simulink subsystem "accelerometer"  (R2023b)
settings: Solver=VariableStepAuto  StartTime=0.0  StopTime=10.0  RelTol=1e-3
undefined symbols (not defined in the file or in its folder): IMU
libraries: sensors_subsystems x5, dyn_lib x1
settings Model: Creator=brent  LastModifiedBy=brent

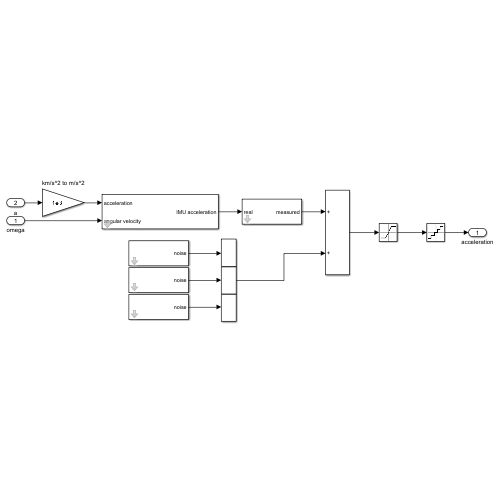
[thumbnail: Simulink's stored preview of the top-level diagram]
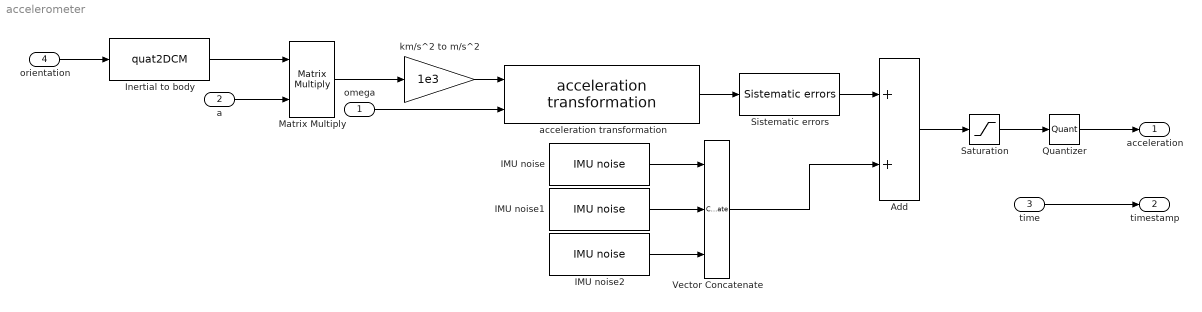
== system accelerometer ==
  omega : Inport
  a : Inport  Port=2
  time : Inport  Port=3
  orientation : Inport  Port=4
  Add : Sum
  IMU noise : sensors_subsystems/IMU noise  data=IMU.accelerometer  arw_seed=abs(round(randn(1)*1e4))  bi_seed=abs(round(randn(1)*1e4))  br_seed=abs(round(randn(1)*1e4))
      settings: SourceProductName=Sensors library
  IMU noise1 : sensors_subsystems/IMU noise  data=IMU.accelerometer  arw_seed=abs(round(randn(1)*1e4))  bi_seed=abs(round(randn(1)*1e4))  br_seed=abs(round(randn(1)*1e4))
      settings: SourceProductName=Sensors library
  IMU noise2 : sensors_subsystems/IMU noise  data=IMU.accelerometer  arw_seed=abs(round(randn(1)*1e4))  bi_seed=abs(round(randn(1)*1e4))  br_seed=abs(round(randn(1)*1e4))
      settings: SourceProductName=Sensors library
  Inertial to body : dyn_lib/quat2DCM
      settings: SourceProductName=Dynamics library
  Matrix Multiply : Product  Multiplication=Matrix(*)
  Quantizer : Quantizer  QuantizationInterval=IMU.accelerometer.resolution.value
  Saturation : Saturate  UpperLimit=IMU.accelerometer.range.value  LowerLimit=-IMU.accelerometer.range.value
  Sistematic errors : sensors_subsystems/Sistematic errors  data=IMU.accelerometer
      settings: SourceProductName=Sensors library
  Vector Concatenate : Concatenate  NumInputs=3
  acceleration transformation : sensors_subsystems/acceleration transformation  pos=IMU.position.value  angles=IMU.orientation.value
      settings: SourceProductName=Sensors library
  km/s^2 to m/s^2 : Gain  Gain=1e3
  acceleration : Outport
  timestamp : Outport  Port=2
  wires:
  omega/1 -> acceleration transformation/2
  Add/1 -> Saturation/1
  Saturation/1 -> Quantizer/1
  Quantizer/1 -> acceleration/1
  acceleration transformation/1 -> Sistematic errors/1
  Sistematic errors/1 -> Add/1
  Vector Concatenate/1 -> Add/2
  km/s^2 to m/s^2/1 -> acceleration transformation/1
  IMU noise2/1 -> Vector Concatenate/3
  IMU noise1/1 -> Vector Concatenate/2
  IMU noise/1 -> Vector Concatenate/1
  time/1 -> timestamp/1
  Inertial to body/1 -> Matrix Multiply/1
  a/1 -> Matrix Multiply/2
  Matrix Multiply/1 -> km/s^2 to m/s^2/1
  orientation/1 -> Inertial to body/1
